simulink model "PID_Controller_Model"  (R2020a)
settings: Solver=VariableStepAuto  StartTime=0.0  StopTime=Sim_Time  MaxStep=0.001  RelTol=1e-3
values from neighbouring files (symbols this model uses):
  b = 10    [PID_Controller_Script.m]
  k = 20    [PID_Controller_Script.m]
  Kd = 50    [PID_Controller_Script.m]
  Ki = 300    [PID_Controller_Script.m]
  Kp = 350    [PID_Controller_Script.m]
  M = 1    [PID_Controller_Script.m]
  Step_value = 1    [PID_Controller_Script.m]
settings Model: Creator=alexd  LastModifiedBy=alexd

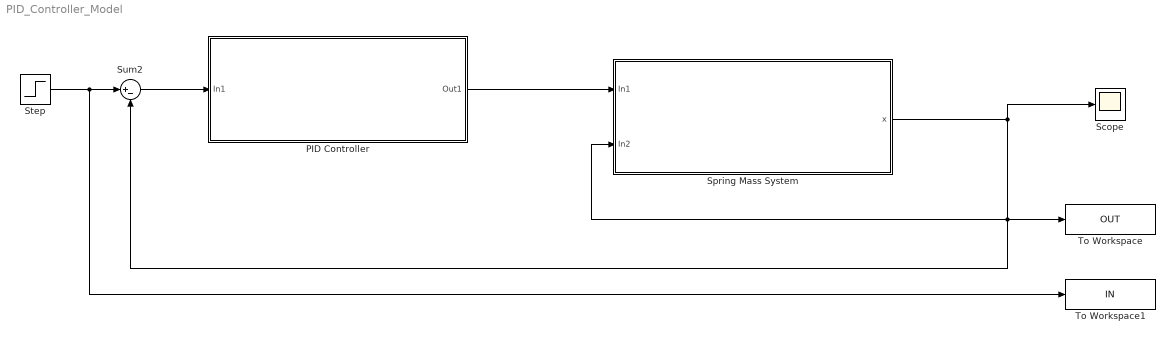
== system PID_Controller_Model ==
  "PID Controller " : Subsystem
  Scope : Scope
  Spring Mass System : Subsystem
  Step : Step  After=Step_value  SampleTime=0
  Sum2 : Sum  Inputs=|+-
  To Workspace : ToWorkspace  VariableName=OUT  SaveFormat=Timeseries  SampleTime=-1
  To Workspace1 : ToWorkspace  VariableName=IN  SaveFormat=Timeseries  SampleTime=-1
  wires:
  Step/1 -> To Workspace1/1, Sum2/1
  Spring Mass System/1(x) -> Spring Mass System/2(In2), Sum2/2, To Workspace/1, Scope/1
  Sum2/1 -> "PID Controller "/1(In1)
  "PID Controller "/1(Out1) -> Spring Mass System/1(In1)

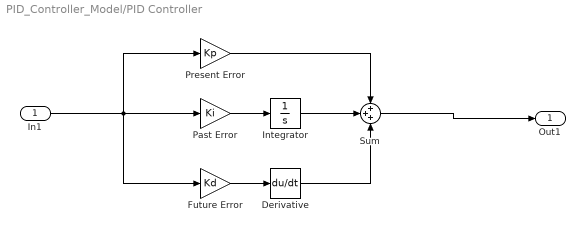
== system PID_Controller_Model/PID Controller  ==
  In1 : Inport
  Derivative : Derivative
  Future Error : Gain  Gain=Kd
  Integrator : Integrator
  Past Error : Gain  Gain=Ki
  Present Error : Gain  Gain=Kp
  Sum : Sum  Inputs=+++
  Out1 : Outport
  wires:
  Sum/1 -> Out1/1
  Integrator/1 -> Sum/2
  In1/1 -> Future Error/1, Past Error/1, Present Error/1
  Future Error/1 -> Derivative/1
  Past Error/1 -> Integrator/1
  Derivative/1 -> Sum/3
  Present Error/1 -> Sum/1

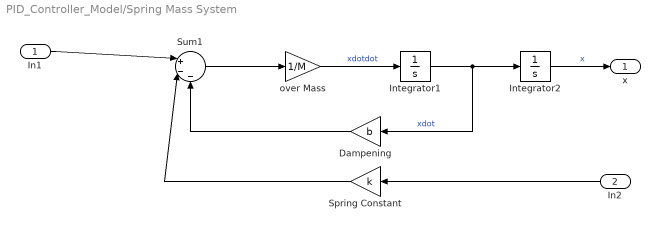
== system PID_Controller_Model/Spring Mass System ==
  In1 : Inport
  In2 : Inport  Port=2
  Dampening : Gain  Gain=b
  Integrator1 : Integrator
  Integrator2 : Integrator
  Spring Constant : Gain  Gain=k
  Sum1 : Sum  Inputs=|+--
  over Mass : Gain  Gain=1/M
  x : Outport
  wires:
  Integrator2/1 -> x/1  "x"
  In2/1 -> Spring Constant/1
  over Mass/1 -> Integrator1/1  "xdotdot"
  In1/1 -> Sum1/1
  Integrator1/1 -> Integrator2/1, Dampening/1  "xdot"
  Dampening/1 -> Sum1/3
  Spring Constant/1 -> Sum1/2
  Sum1/1 -> over Mass/1
